simulink model "Simulacion_NL_final_con_discretizacion"  (R2021a)
settings: Solver=ode15s  StartTime=0.0  StopTime=25  FixedStep=1e-4  MaxStep=1e-4  RelTol=1e-3
undefined symbols (not defined in the file): alpha_cu, ba, beq, Cts, g, Jeq, Ke_i, Ke_theta, Ke_w, ksa, ksia, l_cm, l_l, lambda_m, Ld, Lls, Lq, m, m_l, Pp, r, R0, Rd, Rq, Rs, Rs_REF, Rts_amb, sigbuilder_block, taub_Ts, ts, Ts_REF, wn_i, wn_theta, wsv
libraries: simulink x1
settings Model: Creator=fhlla  LastModifiedBy=rafad

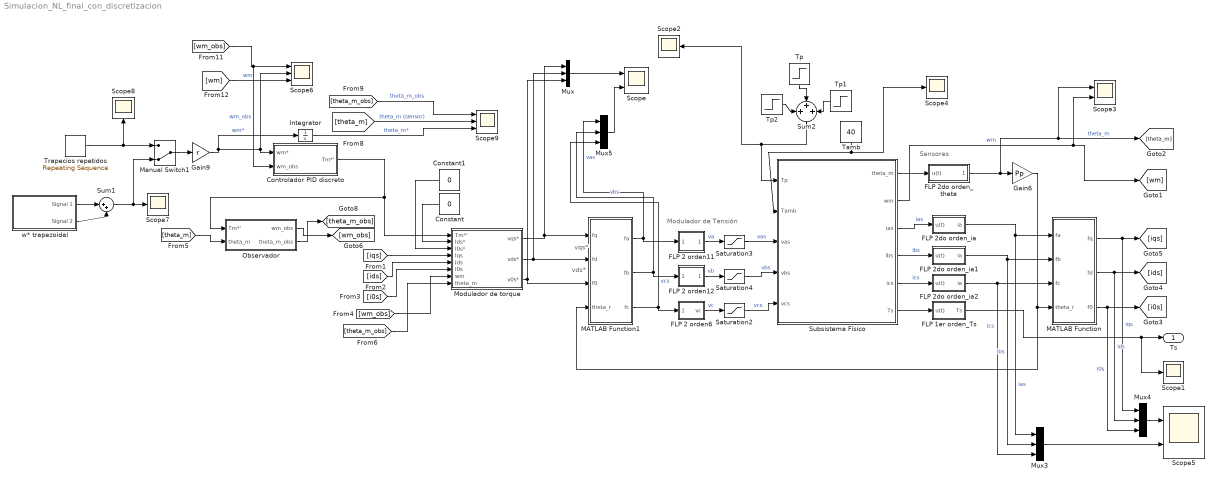
== system Simulacion_NL_final_con_discretizacion ==
  note: vds*
  note: vqs*
  note: Sensores
  note: Modulador de Tensión
  Constant : Constant  Value=0
  Constant1 : Constant  Value=0
  Controlador PID discreto : Subsystem
  FLP 1er orden_Ts : Subsystem
  FLP 2 orden11 : Subsystem
  FLP 2 orden12 : Subsystem
  FLP 2 orden6 : Subsystem
  FLP 2do orden_ia : Subsystem
  FLP 2do orden_ia1 : Subsystem
  FLP 2do orden_ia2 : Subsystem
  FLP 2do orden_theta : Subsystem
  Gain6 : Gain  Gain=Pp
  Gain9 : Gain  Gain=r
  Integrator : Integrator
  MATLAB Function : MATLAB Function  TreatAsAtomicUnit=on
  MATLAB Function1 : MATLAB Function  TreatAsAtomicUnit=on
  Manual Switch1 : ManualSwitch  CurrentSetting=0
  Modulador de torque : Subsystem
  Mux{,3..5} (4 alike) : Mux  Inputs=3
  Observador : Subsystem
  Saturation2 : Saturate  UpperLimit=19.59  LowerLimit=-19.59
  Saturation3 : Saturate  UpperLimit=19.59  LowerLimit=-19.59
  Saturation4 : Saturate  UpperLimit=19.59  LowerLimit=-19.59
  Scope : Scope  NumInputPorts=2
  Scope{1..2,4,7..8} (5 alike) : Scope
  Scope3 : Scope  NumInputPorts=2
  Scope5 : Scope  NumInputPorts=2
  Scope6 : Scope  NumInputPorts=3
  Scope9 : Scope  NumInputPorts=3
  Subsistema Físico : Subsystem
  Sum1 : Sum  Inputs=|++
  Sum2 : Sum  Inputs=+++
  Tamb : Constant  Value=40
  Tp : Step  Time=0.3  After=0  SampleTime=0
  Tp1 : Step  Time=0.5  After=0  SampleTime=0
  Tp2 : Step  Time=0.9  After=0  SampleTime=0
  Trapecios repetidos : simulink/Sources/Repeating Sequence  rep_seq_t=[0 5 5.2 9.8 10 15 15.2 19.8 20]  rep_seq_y=[0 0 1.2566 1.2566 0 0 -1.2566 -1.2566 0]
  w* trapezoidal : Subsystem  Tag=STV Subsys  LoadFcn=sigbuilder_block('load');  StartFcn=sigbuilder_block('start');  StopFcn=sigbuilder_block('stop');  ClipboardFcn=sigbuilder_block('clipboard');  mask(Sigbuilder block){tuvar=[0:10]}
      mask help: Simulink:masks:SigbuilderBlock_MD
      mask init:
      | if ~strcmp(get_param(bdroot(gcbh),'SimulationStatus'),'stopped') tuvar = sigbuilder_block('maskInit'); end
      settings: CopyFcn=sigbuilder_block('copy');  DeleteFcn=sigbuilder_block('delete');  ModelCloseFcn=sigbuilder_block('modelClose');  PreSaveFcn=sigbuilder_block('preSave');  PauseFcn=sigbuilder_block('pause');  ContinueFcn=sigbuilder_block('continue');  NameChangeFcn=sigbuilder_block('namechange');  OpenFcn=sigbuilder_block('open',[6 36 1012.5 435.75 ]);  CloseFcn=sigbuilder_block('close');
      mask Display: plot(0, 0, 100, 100,[2, 2, 32, 32, 2], [68, 8, 8, 68, 68],[32, 2], [38, 38], [32, 19, 2],[53, 60, 44], [32, 17, 17, 2],[16, 16, 31, 31]);txt = getActiveGroup(gcbh);text(2, 100, txt,'verticalAlignment', 'top');
  Ts : Outport
  wires:
  FLP 2do orden_theta/1(theta_m) -> Gain6/1, Scope3/1, [theta_m]  "theta_m"
  Gain6/1 -> MATLAB Function1/4(theta_r), MATLAB Function/4(theta_r)
  FLP 2do orden_ia/1(ia) -> MATLAB Function/1(fa), Mux3/1  "ias"
  FLP 2do orden_ia1/1(ia) -> MATLAB Function/2(fb), Mux3/2  "ibs"
  FLP 2do orden_ia2/1(ia) -> MATLAB Function/3(fc), Mux3/3  "ics"
  MATLAB Function1/1(fa) -> FLP 2 orden11/1(u(t)), Mux5/1  "vas"
  MATLAB Function1/2(fb) -> FLP 2 orden12/1(u(t)), Mux5/2  "vbs"
  MATLAB Function1/3(fc) -> FLP 2 orden6/1(u(t)), Mux5/3  "vcs"
  Tamb/1 -> Subsistema Físico/2(Tamb), Scope4/1
  Subsistema Físico/2(wm) -> [wm], Scope3/2  "wm"
  MATLAB Function/1(fq) -> [iqs], Mux4/1  "iqs"
  MATLAB Function/2(fd) -> [ids], Mux4/2  "ids"
  MATLAB Function/3(f0) -> [i0s], Mux4/3  "i0s"
  FLP 1er orden_Ts/1(Ts) -> Scope1/1, Ts/1
  Mux/1 -> Scope/1
  Tp/1 -> Sum2/2
  Tp2/1 -> Sum2/1
  Tp1/1 -> Sum2/3
  Sum2/1 -> Scope2/1, Subsistema Físico/1(Tp)
  Mux3/1 -> Scope5/2
  Mux4/1 -> Scope5/1
  Mux5/1 -> Scope/2
  Constant/1 -> Modulador de torque/2(Ids*)
  Constant1/1 -> Modulador de torque/3(I0s*)
  Modulador de torque/1(vqs*) -> Mux/1, MATLAB Function1/1(fq)
  Modulador de torque/2(vds*) -> Mux/2, MATLAB Function1/2(fd)
  Modulador de torque/3(v0s*) -> MATLAB Function1/3(f0), Mux/3
  [iqs] -> Modulador de torque/4(Iqs)
  [ids] -> Modulador de torque/5(Ids)
  [i0s] -> Modulador de torque/6(I0s)
  Gain9/1 -> Scope6/2, Controlador PID discreto/1(wm*), Integrator/1  "wm*"
  Sum1/1 -> Manual Switch1/2, Scope7/1
  w* trapezoidal/1(Signal 1) -> Sum1/1
  w* trapezoidal/2(Signal 2) -> Sum1/2
  Manual Switch1/1 -> Gain9/1
  [wm_obs] -> Controlador PID discreto/2(wm_obs), Scope6/1  "wm_obs"
  [wm] -> Scope6/3  "wm"
  [wm_obs] -> Modulador de torque/7(wm)
  [theta_m_obs] -> Modulador de torque/8(theta_m)
  [theta_m] -> Scope9/2  "theta_m (sensor)"
  [theta_m_obs] -> Scope9/1  "theta_m_obs"
  Integrator/1 -> Scope9/3  "theta_m*"
  Subsistema Físico/5(ics) -> FLP 2do orden_ia2/1(u(t))  "ics"
  Subsistema Físico/3(ias) -> FLP 2do orden_ia/1(u(t))  "ias"
  Subsistema Físico/4(ibs) -> FLP 2do orden_ia1/1(u(t))  "ibs"
  Subsistema Físico/6(Ts) -> FLP 1er orden_Ts/1(u(t))
  Subsistema Físico/1(theta_m) -> FLP 2do orden_theta/1(u(t))
  FLP 2 orden11/1(va) -> Saturation3/1  "va"
  Saturation4/1 -> Subsistema Físico/4("vbs ")  "vbs"
  Saturation2/1 -> Subsistema Físico/5("vcs ")  "vcs"
  Saturation3/1 -> Subsistema Físico/3("vas ")  "vas"
  FLP 2 orden6/1(vc) -> Saturation2/1  "vc"
  FLP 2 orden12/1(vb) -> Saturation4/1  "vb"
  Trapecios repetidos/1 -> Scope8/1, Manual Switch1/1
  Controlador PID discreto/1(Tm*') -> Observador/1(Tm*'), Modulador de torque/1(Tm*')
  [theta_m] -> Observador/2(theta_m)
  Observador/1(wm_obs) -> [wm_obs]
  Observador/2(theta_m_obs) -> [theta_m_obs]

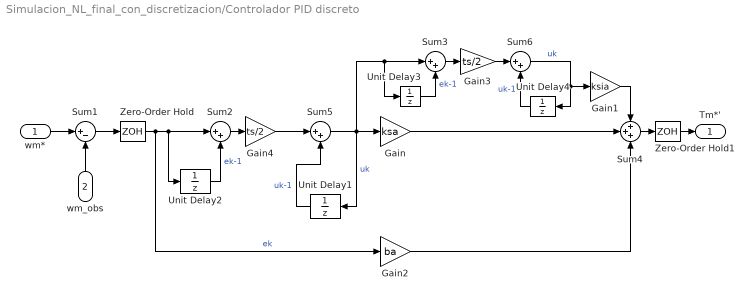
== system Simulacion_NL_final_con_discretizacion/Controlador PID discreto ==
  wm* : Inport
  wm_obs : Inport  Port=2
  Gain : Gain  Gain=ksa
  Gain1 : Gain  Gain=ksia
  Gain2 : Gain  Gain=ba
  Gain3 : Gain  Gain=ts/2
  Gain4 : Gain  Gain=ts/2
  Sum1 : Sum  Inputs=|+-
  Sum{2..3,5..6} (4 alike) : Sum  Inputs=|++
  Sum4 : Sum  Inputs=+++
  Unit Delay{1..4} (4 alike) : UnitDelay  SampleTime=-1  HasFrameUpgradeWarning=on
  Zero-Order Hold : ZeroOrderHold  SampleTime=-1
  Zero-Order Hold1 : ZeroOrderHold  SampleTime=-1
  Tm*' : Outport
  wires:
  Sum1/1 -> Zero-Order Hold/1
  wm_obs/1 -> Sum1/2
  wm*/1 -> Sum1/1
  Zero-Order Hold1/1 -> Tm*'/1
  Zero-Order Hold/1 -> Unit Delay2/1, Sum2/1, Gain2/1  "ek"
  Sum2/1 -> Gain4/1
  Gain1/1 -> Sum4/1
  Sum4/1 -> Zero-Order Hold1/1
  Gain/1 -> Sum4/2
  Gain2/1 -> Sum4/3
  Unit Delay2/1 -> Sum2/2  "ek-1"
  Sum5/1 -> Gain/1, Unit Delay3/1, Sum3/1, Unit Delay1/1  "uk"
  Gain4/1 -> Sum5/1
  Unit Delay1/1 -> Sum5/2  "uk-1"
  Unit Delay3/1 -> Sum3/2  "ek-1"
  Sum3/1 -> Gain3/1
  Gain3/1 -> Sum6/1
  Unit Delay4/1 -> Sum6/2  "uk-1"
  Sum6/1 -> Gain1/1, Unit Delay4/1  "uk"

== system Simulacion_NL_final_con_discretizacion/FLP 1er orden_Ts ==
  u(t) : Inport
  Gain : Gain  Gain=1/taub_Ts
  Gain1 : Gain  Gain=1/taub_Ts
  Integrator1 : Integrator  InitialCondition=40
  Sum : Sum  Inputs=|+|-
  Ts : Outport
  wires:
  u(t)/1 -> Gain/1
  Integrator1/1 -> Ts/1, Gain1/1  "x1"
  Gain/1 -> Sum/1
  Gain1/1 -> Sum/2
  Sum/1 -> Integrator1/1  "d(x1)"

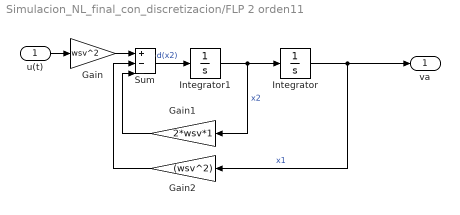
== system Simulacion_NL_final_con_discretizacion/FLP 2 orden11 ==
  u(t) : Inport
  Gain : Gain  Gain=wsv^2
  Gain1 : Gain  Gain=2*wsv*1
  Gain2 : Gain  Gain=(wsv^2)
  Integrator : Integrator
  Integrator1 : Integrator
  Sum : Sum  Inputs=|+|-|-
  va : Outport
  wires:
  u(t)/1 -> Gain/1
  Integrator1/1 -> Gain1/1, Integrator/1  "x2"
  Integrator/1 -> Gain2/1, va/1  "x1"
  Gain/1 -> Sum/1
  Sum/1 -> Integrator1/1  "d(x2)"
  Gain1/1 -> Sum/3
  Gain2/1 -> Sum/2

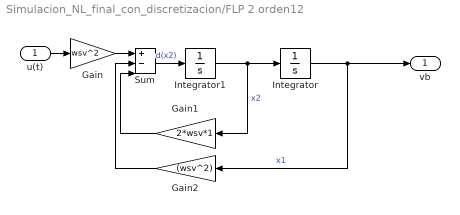
== system Simulacion_NL_final_con_discretizacion/FLP 2 orden12 ==
  u(t) : Inport
  Gain : Gain  Gain=wsv^2
  Gain1 : Gain  Gain=2*wsv*1
  Gain2 : Gain  Gain=(wsv^2)
  Integrator : Integrator
  Integrator1 : Integrator
  Sum : Sum  Inputs=|+|-|-
  vb : Outport
  wires:
  u(t)/1 -> Gain/1
  Integrator1/1 -> Gain1/1, Integrator/1  "x2"
  Integrator/1 -> Gain2/1, vb/1  "x1"
  Gain/1 -> Sum/1
  Sum/1 -> Integrator1/1  "d(x2)"
  Gain1/1 -> Sum/3
  Gain2/1 -> Sum/2

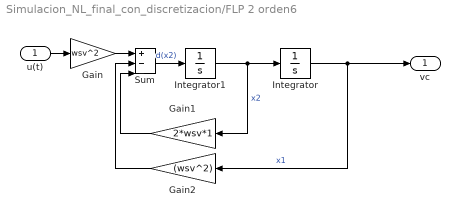
== system Simulacion_NL_final_con_discretizacion/FLP 2 orden6 ==
  u(t) : Inport
  Gain : Gain  Gain=wsv^2
  Gain1 : Gain  Gain=2*wsv*1
  Gain2 : Gain  Gain=(wsv^2)
  Integrator : Integrator
  Integrator1 : Integrator
  Sum : Sum  Inputs=|+|-|-
  vc : Outport
  wires:
  u(t)/1 -> Gain/1
  Integrator1/1 -> Gain1/1, Integrator/1  "x2"
  Integrator/1 -> Gain2/1, vc/1  "x1"
  Gain/1 -> Sum/1
  Sum/1 -> Integrator1/1  "d(x2)"
  Gain1/1 -> Sum/3
  Gain2/1 -> Sum/2

== system Simulacion_NL_final_con_discretizacion/FLP 2do orden_ia ==
  u(t) : Inport
  Gain : Gain  Gain=wn_i^2
  Gain1 : Gain  Gain=2*wn_i*1
  Gain2 : Gain  Gain=(wn_i^2)
  Integrator : Integrator
  Integrator1 : Integrator
  Sum : Sum  Inputs=|+|-|-
  ia : Outport
  wires:
  u(t)/1 -> Gain/1
  Integrator1/1 -> Gain1/1, Integrator/1  "x2"
  Integrator/1 -> Gain2/1, ia/1  "x1"
  Gain/1 -> Sum/1
  Sum/1 -> Integrator1/1  "d(x2)"
  Gain1/1 -> Sum/3
  Gain2/1 -> Sum/2

== system Simulacion_NL_final_con_discretizacion/FLP 2do orden_ia1 ==
  u(t) : Inport
  Gain : Gain  Gain=wn_i^2
  Gain1 : Gain  Gain=2*wn_i*1
  Gain2 : Gain  Gain=(wn_i^2)
  Integrator : Integrator
  Integrator1 : Integrator
  Sum : Sum  Inputs=|+|-|-
  ia : Outport
  wires:
  u(t)/1 -> Gain/1
  Integrator1/1 -> Gain1/1, Integrator/1  "x2"
  Integrator/1 -> Gain2/1, ia/1  "x1"
  Gain/1 -> Sum/1
  Sum/1 -> Integrator1/1  "d(x2)"
  Gain1/1 -> Sum/3
  Gain2/1 -> Sum/2

== system Simulacion_NL_final_con_discretizacion/FLP 2do orden_ia2 ==
  u(t) : Inport
  Gain : Gain  Gain=wn_i^2
  Gain1 : Gain  Gain=2*wn_i*1
  Gain2 : Gain  Gain=(wn_i^2)
  Integrator : Integrator
  Integrator1 : Integrator
  Sum : Sum  Inputs=|+|-|-
  ia : Outport
  wires:
  u(t)/1 -> Gain/1
  Integrator1/1 -> Gain1/1, Integrator/1  "x2"
  Integrator/1 -> Gain2/1, ia/1  "x1"
  Gain/1 -> Sum/1
  Sum/1 -> Integrator1/1  "d(x2)"
  Gain1/1 -> Sum/3
  Gain2/1 -> Sum/2

== system Simulacion_NL_final_con_discretizacion/FLP 2do orden_theta ==
  u(t) : Inport
  Gain : Gain  Gain=wn_theta^2
  Gain1 : Gain  Gain=2*wn_theta*1
  Gain2 : Gain  Gain=(wn_theta^2)
  Integrator : Integrator
  Integrator1 : Integrator
  Sum : Sum  Inputs=|+|-|-
  theta_m : Outport
  wires:
  u(t)/1 -> Gain/1
  Integrator1/1 -> Gain1/1, Integrator/1  "x2"
  Integrator/1 -> Gain2/1, theta_m/1  "x1"
  Gain/1 -> Sum/1
  Sum/1 -> Integrator1/1  "d(x2)"
  Gain1/1 -> Sum/3
  Gain2/1 -> Sum/2

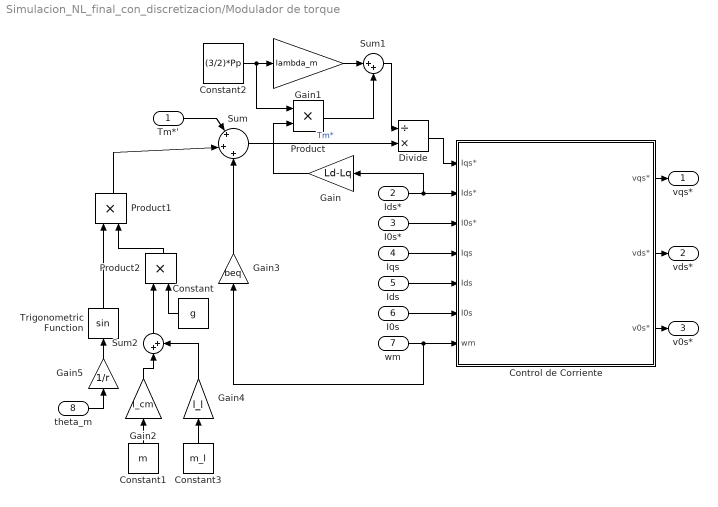
== system Simulacion_NL_final_con_discretizacion/Modulador de torque ==
  Tm*' : Inport
  Ids* : Inport  Port=2
  I0s* : Inport  Port=3
  Iqs : Inport  Port=4
  Ids : Inport  Port=5
  I0s : Inport  Port=6
  wm : Inport  Port=7
  theta_m : Inport  Port=8
  Constant : Constant  Value=g
  Constant1 : Constant  Value=m
  Constant2 : Constant  Value=(3/2)*Pp
  Constant3 : Constant  Value=m_l
  Control de Corriente : Subsystem
  Divide : Product  Inputs=/*
  Gain : Gain  Gain=Ld-Lq
  Gain1 : Gain  Gain=lambda_m
  Gain2 : Gain  Gain=l_cm
  Gain3 : Gain  Gain=beq
  Gain4 : Gain  Gain=l_l
  Gain5 : Gain  Gain=1/r
  Product : Product
  Product1 : Product
  Product2 : Product
  Sum : Sum  Inputs=|+|+|+
  Sum1 : Sum  Inputs=|++
  Sum2 : Sum  Inputs=|++
  Trigonometric Function : Trigonometry
  vqs* : Outport
  vds* : Outport  Port=2
  v0s* : Outport  Port=3
  wires:
  Product/1 -> Sum1/2
  I0s/1 -> Control de Corriente/6(I0s)
  Control de Corriente/2(vds*) -> vds*/1
  Divide/1 -> Control de Corriente/1(Iqs*)
  Sum/1 -> Divide/2  "Tm*"
  I0s*/1 -> Control de Corriente/3(I0s*)
  Control de Corriente/3(v0s*) -> v0s*/1
  wm/1 -> Gain3/1, Control de Corriente/7(wm)
  Constant2/1 -> Gain1/1, Product/1
  Ids*/1 -> Gain/1, Control de Corriente/2(Ids*)
  Ids/1 -> Control de Corriente/5(Ids)
  Gain/1 -> Product/2
  Iqs/1 -> Control de Corriente/4(Iqs)
  Control de Corriente/1(vqs*) -> vqs*/1
  Tm*'/1 -> Sum/1
  Gain1/1 -> Sum1/1
  Sum1/1 -> Divide/1
  Constant1/1 -> Gain2/1
  Constant3/1 -> Gain4/1
  Gain5/1 -> Trigonometric Function/1
  Gain2/1 -> Sum2/1
  Gain4/1 -> Sum2/2
  Sum2/1 -> Product2/1
  Constant/1 -> Product2/2
  theta_m/1 -> Gain5/1
  Trigonometric Function/1 -> Product1/1
  Product2/1 -> Product1/2
  Gain3/1 -> Sum/3
  Product1/1 -> Sum/2

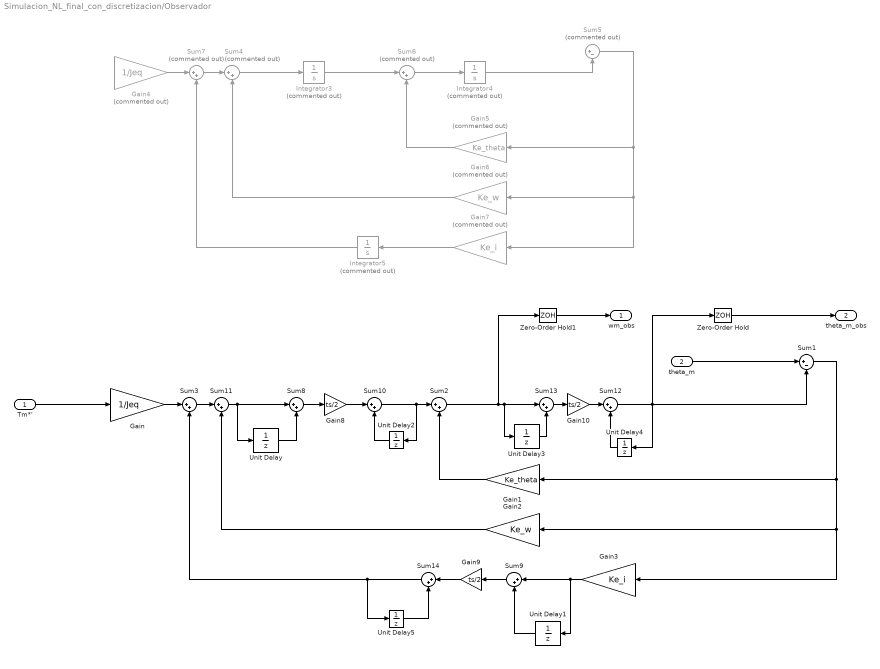
== system Simulacion_NL_final_con_discretizacion/Observador ==
  Tm*' : Inport
  theta_m : Inport  Port=2
  Gain : Gain  Gain=1/Jeq
  Gain1 : Gain  Gain=Ke_theta
  Gain10 : Gain  Gain=ts/2
  Gain2 : Gain  Gain=Ke_w
  Gain3 : Gain  Gain=Ke_i
  Gain4 : Gain  Commented=on  Gain=1/Jeq
  Gain5 : Gain  Commented=on  Gain=Ke_theta
  Gain6 : Gain  Commented=on  Gain=Ke_w
  Gain7 : Gain  Commented=on  Gain=Ke_i
  Gain8 : Gain  Gain=ts/2
  Gain9 : Gain  Gain=ts/2
  Integrator3 : Integrator  Commented=on
  Integrator4 : Integrator  Commented=on
  Integrator5 : Integrator  Commented=on
  Sum1 : Sum  Inputs=|+-
  Sum{2..3,8..14} (9 alike) : Sum  Inputs=|++
  Sum4 : Sum  Commented=on  Inputs=|++
  Sum5 : Sum  Commented=on  Inputs=|+-
  Sum6 : Sum  Commented=on  Inputs=|++
  Sum7 : Sum  Commented=on  Inputs=|++
  Unit Delay{,1..5} (6 alike) : UnitDelay  SampleTime=-1  HasFrameUpgradeWarning=on
  Zero-Order Hold : ZeroOrderHold  SampleTime=-1
  Zero-Order Hold1 : ZeroOrderHold  SampleTime=-1
  wm_obs : Outport
  theta_m_obs : Outport  Port=2
  wires:
  Gain1/1 -> Sum2/2
  Sum1/1 -> Gain1/1, Gain3/1, Gain2/1
  Sum6/1 -> Integrator4/1
  Integrator5/1 -> Sum7/2
  Sum4/1 -> Integrator3/1
  Sum5/1 -> Gain7/1, Gain6/1, Gain5/1
  Integrator3/1 -> Sum6/1
  Gain7/1 -> Integrator5/1
  Integrator4/1 -> Sum5/2
  Gain6/1 -> Sum4/2
  Sum7/1 -> Sum4/1
  Gain5/1 -> Sum6/2
  Gain4/1 -> Sum7/1
  Gain/1 -> Sum3/1
  Tm*'/1 -> Gain/1
  Sum2/1 -> Sum13/1, Unit Delay3/1, Zero-Order Hold1/1
  Gain2/1 -> Sum11/2
  Sum3/1 -> Sum11/1
  Sum8/1 -> Gain8/1
  Sum11/1 -> Unit Delay/1, Sum8/1
  theta_m/1 -> Sum1/1
  Zero-Order Hold/1 -> theta_m_obs/1
  Zero-Order Hold1/1 -> wm_obs/1
  Unit Delay/1 -> Sum8/2
  Gain8/1 -> Sum10/1
  Sum10/1 -> Unit Delay2/1, Sum2/1
  Unit Delay2/1 -> Sum10/2
  Unit Delay3/1 -> Sum13/2
  Sum13/1 -> Gain10/1
  Gain10/1 -> Sum12/1
  Unit Delay4/1 -> Sum12/2
  Sum12/1 -> Zero-Order Hold/1, Unit Delay4/1, Sum1/2
  Gain3/1 -> Unit Delay1/1, Sum9/1
  Unit Delay1/1 -> Sum9/2
  Sum9/1 -> Gain9/1
  Gain9/1 -> Sum14/1
  Unit Delay5/1 -> Sum14/2
  Sum14/1 -> Unit Delay5/1, Sum3/2

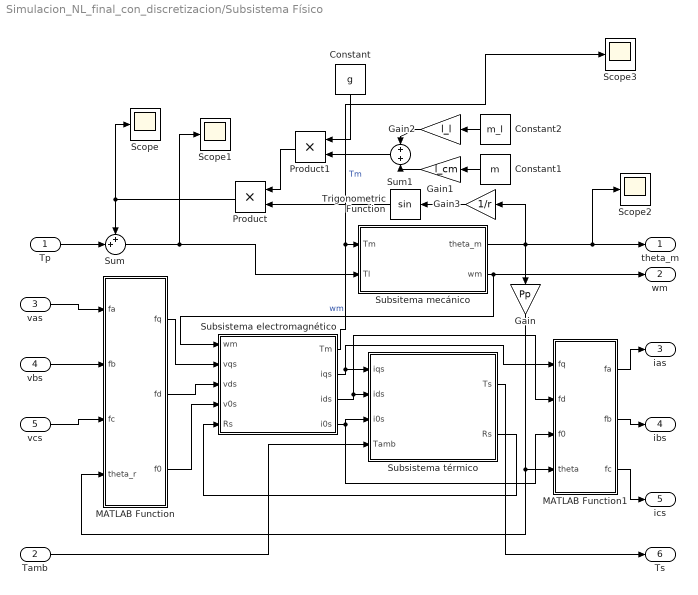
== system Simulacion_NL_final_con_discretizacion/Subsistema Físico ==
  Tp : Inport
  Tamb : Inport  Port=2
  "vas " : Inport  Port=3
  "vbs " : Inport  Port=4
  "vcs " : Inport  Port=5
  Constant : Constant  Value=g
  Constant1 : Constant  Value=m
  Constant2 : Constant  Value=m_l
  Gain : Gain  Gain=Pp
  Gain1 : Gain  Gain=l_cm
  Gain2 : Gain  Gain=l_l
  Gain3 : Gain  Gain=1/r
  MATLAB Function : MATLAB Function  TreatAsAtomicUnit=on
  MATLAB Function1 : MATLAB Function  TreatAsAtomicUnit=on
  Product : Product
  Product1 : Product
  Scope{,1..3} (4 alike) : Scope
  Subsistema electromagnético : Subsystem
  Subsistema térmico : Subsystem
  Subsitema mecánico : Subsystem
  Sum : Sum  Inputs=++|
  Sum1 : Sum  Inputs=+|+
  Trigonometric Function : Trigonometry
  theta_m : Outport
  wm : Outport  Port=2
  ias : Outport  Port=3
  ibs : Outport  Port=4
  ics : Outport  Port=5
  Ts : Outport  Port=6
  wires:
  Constant/1 -> Product1/1
  Trigonometric Function/1 -> Product/2
  Sum1/1 -> Product1/2
  Constant1/1 -> Gain1/1
  Product1/1 -> Product/1
  Product/1 -> Scope/1, Sum/1
  Gain1/1 -> Sum1/2
  Sum/1 -> Scope1/1, Subsitema mecánico/2(Tl)
  Tp/1 -> Sum/2
  Subsistema electromagnético/4(i0s) -> MATLAB Function1/3(f0), Subsistema térmico/3(i0s)
  MATLAB Function1/2(fb) -> ibs/1
  "vcs "/1 -> MATLAB Function/3(fc)
  Subsistema electromagnético/1(Tm) -> Scope3/1, Subsitema mecánico/1(Tm)  "Tm"
  MATLAB Function1/1(fa) -> ias/1
  MATLAB Function/2(fd) -> Subsistema electromagnético/3(vds)
  Tamb/1 -> Subsistema térmico/4(Tamb)
  Subsistema térmico/1(Ts) -> Ts/1
  MATLAB Function/3(f0) -> Subsistema electromagnético/4(v0s)
  Gain2/1 -> Sum1/1
  MATLAB Function1/3(fc) -> ics/1
  Subsitema mecánico/1(theta_m) -> Gain3/1, Scope2/1, theta_m/1, Gain/1
  Gain/1 -> MATLAB Function/4(theta_r), MATLAB Function1/4(theta)
  Subsistema electromagnético/2(iqs) -> MATLAB Function1/1(fq), Subsistema térmico/1(iqs)
  Subsistema electromagnético/3(ids) -> MATLAB Function1/2(fd), Subsistema térmico/2(ids)
  "vbs "/1 -> MATLAB Function/2(fb)
  Subsitema mecánico/2(wm) -> wm/1, Subsistema electromagnético/1(wm)  "wm"
  Constant2/1 -> Gain2/1
  MATLAB Function/1(fq) -> Subsistema electromagnético/2(vqs)
  Gain3/1 -> Trigonometric Function/1
  Subsistema térmico/2(Rs) -> Subsistema electromagnético/5(Rs)
  "vas "/1 -> MATLAB Function/1(fa)

== system Simulacion_NL_final_con_discretizacion/w* trapezoidal ==
  Demux : Demux  Tag=STV Demux  Outputs=2
      settings: DisplayOption=none
  FromWs : FromWorkspace  Tag=STV FromWs  VariableName=tuvar
      SigBuilderData=|
      | common.afterFinalStr = 'Extrapolate'
      | common.sampleTime = 0
      | dataSet.timeRange = [0 25]
      | dataSet.name = 'Group 1'
      | sbobj.Groups.Name = 'Group 1'
      | sbobj.Groups.Signals(1).Name = 'Signal 1'
      | sbobj.Groups.Signals(1).XData = [0 5 5.2 9.8 10 25]
      | sbobj.Groups.Signals(1).YData = [0 0 1.25663706144 1.25663706144 0 0]
      | sbobj.Groups.Signals(2).Name = 'Signal 2'
      | sbobj.Groups.Signals(2).XData = [0 15 15.2 19.8 20 25]
      | sbobj.Groups.Signals(2).YData = [0 0 -1.25663706144 -1.25663706144 0 0]
      | sbobj.Groups.TimeRange = [0 25]
  Signal 1 : Outport  Tag=STV Outport
  Signal 2 : Outport  Tag=STV Outport  Port=2
  wires:
  FromWs/1 -> Demux/1
  Demux/1 -> Signal 1/1
  Demux/2 -> Signal 2/1

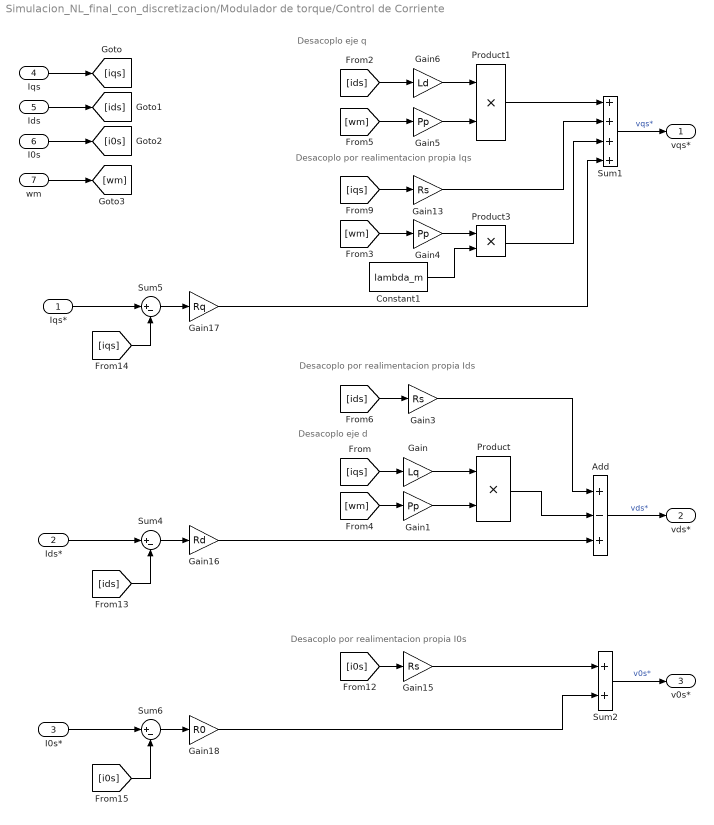
== system Simulacion_NL_final_con_discretizacion/Modulador de torque/Control de Corriente ==
  note: Desacoplo por realimentacion propia I0s
  note: Desacoplo por realimentacion propia Iqs
  note: Desacoplo por realimentacion propia Ids
  note: Desacoplo eje d
  note: Desacoplo eje q
  Iqs* : Inport
  Ids* : Inport  Port=2
  I0s* : Inport  Port=3
  Iqs : Inport  Port=4
  Ids : Inport  Port=5
  I0s : Inport  Port=6
  wm : Inport  Port=7
  Add : Sum  Inputs=+-+
  Constant1 : Constant  Value=lambda_m
  Gain : Gain  Gain=Lq
  Gain1 : Gain  Gain=Pp
  Gain13 : Gain  Gain=Rs
  Gain15 : Gain  Gain=Rs
  Gain16 : Gain  Gain=Rd
  Gain17 : Gain  Gain=Rq
  Gain18 : Gain  Gain=R0
  Gain3 : Gain  Gain=Rs
  Gain4 : Gain  Gain=Pp
  Gain5 : Gain  Gain=Pp
  Gain6 : Gain  Gain=Ld
  Product : Product
  Product1 : Product
  Product3 : Product
  Sum1 : Sum  Inputs=++++
  Sum2 : Sum
  Sum4 : Sum  Inputs=|+-
  Sum5 : Sum  Inputs=|+-
  Sum6 : Sum  Inputs=|+-
  vqs* : Outport
  vds* : Outport  Port=2
  v0s* : Outport  Port=3
  wires:
  [i0s] -> Sum6/2
  Sum2/1 -> v0s*/1  "v0s*"
  Iqs*/1 -> Sum5/1
  I0s*/1 -> Sum6/1
  [iqs] -> Gain13/1
  [ids] -> Sum4/2
  [i0s] -> Gain15/1
  Sum5/1 -> Gain17/1
  [iqs] -> Sum5/2
  [ids] -> Gain3/1
  Gain13/1 -> Sum1/2
  Sum6/1 -> Gain18/1
  Ids*/1 -> Sum4/1
  Gain15/1 -> Sum2/1
  Gain18/1 -> Sum2/2
  Gain17/1 -> Sum1/4
  Product1/1 -> Sum1/1
  Product/1 -> Add/2
  Gain5/1 -> Product1/2
  Gain/1 -> Product/1
  Gain4/1 -> Product3/1
  Sum4/1 -> Gain16/1
  Constant1/1 -> Product3/2
  Product3/1 -> Sum1/3
  Add/1 -> vds*/1  "vds*"
  Sum1/1 -> vqs*/1  "vqs*"
  Iqs/1 -> [iqs]
  Ids/1 -> [ids]
  I0s/1 -> [i0s]
  [iqs] -> Gain/1
  Gain1/1 -> Product/2
  [wm] -> Gain1/1
  wm/1 -> [wm]
  [wm] -> Gain4/1
  [wm] -> Gain5/1
  [ids] -> Gain6/1
  Gain6/1 -> Product1/1
  Gain16/1 -> Add/3
  Gain3/1 -> Add/1

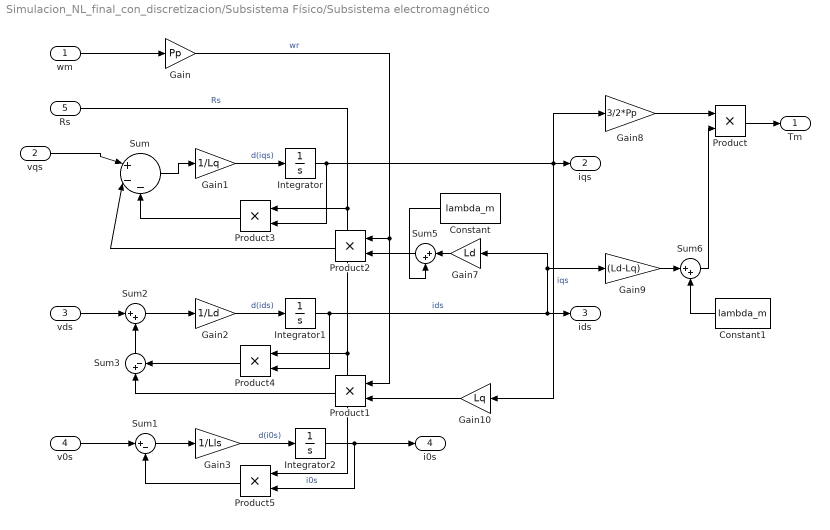
== system Simulacion_NL_final_con_discretizacion/Subsistema Físico/Subsistema electromagnético ==
  wm : Inport
  vqs : Inport  Port=2
  vds : Inport  Port=3
  v0s : Inport  Port=4
  Rs : Inport  Port=5
  Constant : Constant  Value=lambda_m
  Constant1 : Constant  Value=lambda_m
  Gain : Gain  Gain=Pp
  Gain1 : Gain  Gain=1/Lq
  Gain10 : Gain  Gain=Lq
  Gain2 : Gain  Gain=1/Ld
  Gain3 : Gain  Gain=1/Lls
  Gain7 : Gain  Gain=Ld
  Gain8 : Gain  Gain=3/2*Pp
  Gain9 : Gain  Gain=(Ld-Lq)
  Integrator : Integrator
  Integrator1 : Integrator  InitialCondition=0.5
  Integrator2 : Integrator
  Product{,1..5} (6 alike) : Product
  Sum : Sum  Inputs=|+--
  Sum1 : Sum  Inputs=|+-
  Sum2 : Sum  Inputs=|++
  Sum3 : Sum  Inputs=|+-
  Sum5 : Sum  Inputs=|++
  Sum6 : Sum  Inputs=|++
  Tm : Outport
  iqs : Outport  Port=2
  ids : Outport  Port=3
  i0s : Outport  Port=4
  wires:
  Gain7/1 -> Sum5/1
  Sum1/1 -> Gain3/1
  Integrator1/1 -> Product4/2, Gain9/1, Gain7/1, ids/1  "ids"
  Product5/1 -> Sum1/2
  Gain/1 -> Product2/1, Product1/1  "wr"
  Product/1 -> Tm/1
  v0s/1 -> Sum1/1
  Gain9/1 -> Sum6/1
  Gain8/1 -> Product/1
  Sum5/1 -> Product2/2
  Gain1/1 -> Integrator/1  "d(iqs)"
  Constant/1 -> Sum5/2
  Integrator2/1 -> Product5/2, i0s/1  "i0s"
  Gain10/1 -> Product1/2
  Sum/1 -> Gain1/1
  Integrator/1 -> Product3/2, Gain10/1, Gain8/1, iqs/1  "iqs"
  vds/1 -> Sum2/1
  Constant1/1 -> Sum6/2
  Gain2/1 -> Integrator1/1  "d(ids)"
  Gain3/1 -> Integrator2/1  "d(i0s)"
  Product1/1 -> Sum3/1
  Sum2/1 -> Gain2/1
  Sum3/1 -> Sum2/2
  vqs/1 -> Sum/1
  Sum6/1 -> Product/2
  wm/1 -> Gain/1
  Product4/1 -> Sum3/2
  Rs/1 -> Product3/1, Product5/1, Product4/1  "Rs"
  Product3/1 -> Sum/3
  Product2/1 -> Sum/2

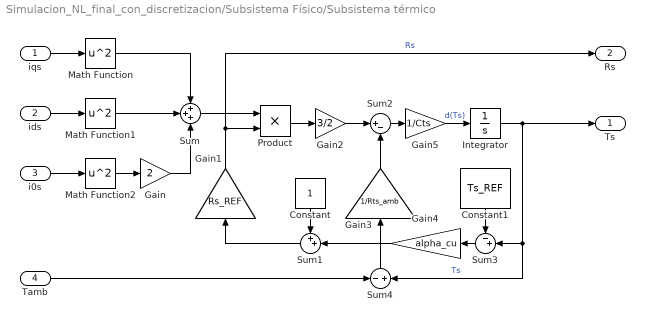
== system Simulacion_NL_final_con_discretizacion/Subsistema Físico/Subsistema térmico ==
  iqs : Inport
  ids : Inport  Port=2
  i0s : Inport  Port=3
  Tamb : Inport  Port=4
  Constant : Constant
  Constant1 : Constant  Value=Ts_REF
  Gain : Gain  Gain=2
  Gain1 : Gain  Gain=Rs_REF
  Gain2 : Gain  Gain=3/2
  Gain3 : Gain  Gain=1/Rts_amb
  Gain4 : Gain  Gain=alpha_cu
  Gain5 : Gain  Gain=1/Cts
  Integrator : Integrator  InitialCondition=40
  Math Function : Math  Operator=square  SaturateOnIntegerOverflow=on
  Math Function1 : Math  Operator=square  SaturateOnIntegerOverflow=on
  Math Function2 : Math  Operator=square  SaturateOnIntegerOverflow=on
  Product : Product
  Sum : Sum  Inputs=+++
  Sum1 : Sum  Inputs=++|
  Sum2 : Sum  Inputs=|+-
  Sum3 : Sum  Inputs=-+|
  Sum4 : Sum  Inputs=-|+
  Ts : Outport
  Rs : Outport  Port=2
  wires:
  Sum/1 -> Product/1
  Tamb/1 -> Sum4/1
  Gain3/1 -> Sum2/2
  Sum1/1 -> Gain1/1
  Product/1 -> Gain2/1
  Integrator/1 -> Ts/1, Sum3/2, Sum4/2  "Ts"
  iqs/1 -> Math Function/1
  Gain5/1 -> Integrator/1  "d(Ts)"
  Sum2/1 -> Gain5/1
  Gain1/1 -> Rs/1, Product/2  "Rs"
  Constant/1 -> Sum1/1
  Gain/1 -> Sum/3
  ids/1 -> Math Function1/1
  i0s/1 -> Math Function2/1
  Gain2/1 -> Sum2/1
  Math Function1/1 -> Sum/2
  Sum4/1 -> Gain3/1
  Math Function2/1 -> Gain/1
  Math Function/1 -> Sum/1
  Constant1/1 -> Sum3/1
  Gain4/1 -> Sum1/2
  Sum3/1 -> Gain4/1

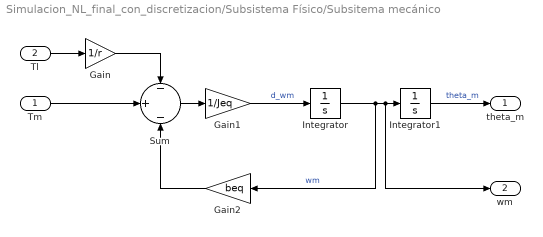
== system Simulacion_NL_final_con_discretizacion/Subsistema Físico/Subsitema mecánico ==
  Tm : Inport
  Tl : Inport  Port=2
  Gain : Gain  Gain=1/r
  Gain1 : Gain  Gain=1/Jeq
  Gain2 : Gain  Gain=beq
  Integrator : Integrator
  Integrator1 : Integrator
  Sum : Sum  Inputs=-|+|-
  theta_m : Outport
  wm : Outport  Port=2
  wires:
  Integrator1/1 -> theta_m/1  "theta_m"
  Tl/1 -> Gain/1
  Gain/1 -> Sum/1
  Sum/1 -> Gain1/1
  Gain1/1 -> Integrator/1  "d_wm"
  Tm/1 -> Sum/2
  Gain2/1 -> Sum/3
  Integrator/1 -> Gain2/1, wm/1, Integrator1/1  "wm"

== matlab function Simulacion_NL_final_con_discretizacion/MATLAB Function1 ==
  data: fq input; fa output; fd input; f0 input; theta_r input; fb output; fc output
function [fa,fb,fc] = TI_Park(fq,fd,f0,theta_r)
f = [        cos(theta_r)          sin(theta_r)        1;
     cos(theta_r - (2*pi)/3) sin(theta_r - (2*pi)/3)   1;
     cos(theta_r + (2*pi)/3) sin(theta_r + (2*pi)/3)   1];

resultados = f*[fq;fd;f0];
fa = resultados(1);
fb = resultados(2);
fc = resultados(3);

== matlab function Simulacion_NL_final_con_discretizacion/MATLAB Function ==
  data: fa input; fq output; fb input; fc input; theta_r input; fd output; f0 output
function [fq, fd, f0] = TD_Park(fa, fb, fc, theta_r)
    f = (2/3) * [cos(theta_r)               cos(theta_r - (2*pi)/3)      cos(theta_r + (2*pi)/3);
                 sin(theta_r)               sin(theta_r - (2*pi)/3)      sin(theta_r + (2*pi)/3);
                 1/2                      1/2                        1/2                   ];

    resultados = f * [fa; fb; fc];
    fq = resultados(1);
    fd = resultados(2);
    f0 = resultados(3);
end

== matlab function Simulacion_NL_final_con_discretizacion/Subsistema Físico/MATLAB Function1 ==
  data: fq input; fa output; fd input; f0 input; theta input; fb output; fc output
function [fa,fb,fc] = TI_Park(fq,fd,f0,theta)
f = [        cos(theta)          sin(theta)        1;
     cos(theta - (2*pi)/3) sin(theta - (2*pi)/3)   1;
     cos(theta + (2*pi)/3) sin(theta + (2*pi)/3)   1];

resultados = f*[fq;fd;f0];
fa = resultados(1);
fb = resultados(2);
fc = resultados(3);

== matlab function Simulacion_NL_final_con_discretizacion/Subsistema Físico/MATLAB Function ==
  data: fa input; fq output; fb input; fc input; theta_r input; fd output; f0 output
function [fq, fd, f0] = TD_Park(fa, fb, fc, theta_r)
    f = (2/3) * [cos(theta_r)               cos(theta_r - (2*pi)/3)      cos(theta_r + (2*pi)/3);
                 sin(theta_r)               sin(theta_r - (2*pi)/3)      sin(theta_r + (2*pi)/3);
                 1/2                      1/2                        1/2                   ];

    resultados = f * [fa; fb; fc];
    fq = resultados(1);
    fd = resultados(2);
    f0 = resultados(3);
end
